simulink model "V1_Pendel"  (R2021a)
settings: Solver=ode3  StartTime=0.0  StopTime=Zeit(end)  FixedStep=0.001  RelTol=1e-3
values from neighbouring files (symbols this model uses):
  Amplitude_rad = (Amplitude/180) * pi    [V1_Schaetzung_d.m]
  d = 0.0042    [V1_Parameter_Stahl_math.m]    (also in V1_Parameter_Stahl_phys.m = 0.0043; V1_Parameter_Styropor_math.m = 0.00019; V1_Parameter_Styropor_phys.m = 0.0018; V1_Schaetzung_d.m = m*g*l*(cos(phi_2) - cos(phi_1))/Integral)
  g = 9.81    [V1_Parameter_Stahl_math.m]    (also in V1_Parameter_Stahl_phys.m; V1_Parameter_Styropor_math.m; V1_Parameter_Styropor_phys.m)
  J = m * l^2    (= 0.503397949)    [V1_Parameter_Stahl_math.m]    (also in V1_Parameter_Stahl_phys.m = 0.512724514275; V1_Parameter_Styropor_math.m = 0.00169341029375; V1_Parameter_Styropor_phys.m = 0.0103382057863)
  l = l_S - s + r_K    (= 0.6005)    [V1_Parameter_Stahl_math.m]    (also in V1_Parameter_Stahl_phys.m = 0.459355833378; V1_Parameter_Styropor_math.m = 0.60025; V1_Parameter_Styropor_phys.m = 0.0522765339967)
  m = m_K    (= 1.396)    [V1_Parameter_Stahl_math.m]    (also in V1_Parameter_Stahl_phys.m = 1.8737; V1_Parameter_Styropor_math.m = 0.0047; V1_Parameter_Styropor_phys.m = 0.4824)
settings Model: Creator=schmi  LastModifiedBy=schmi

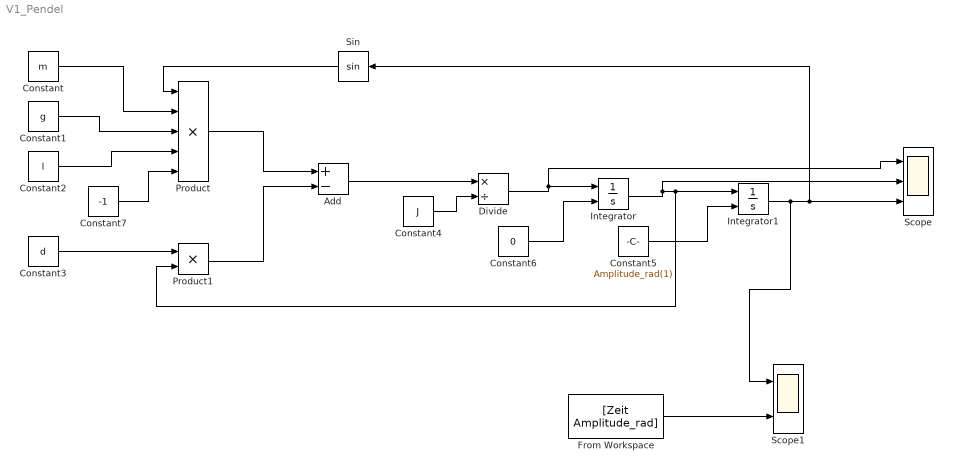
== system V1_Pendel ==
  Add : Sum  Inputs=+-
  Constant : Constant  Value=m
  Constant1 : Constant  Value=g
  Constant2 : Constant  Value=l
  Constant3 : Constant  Value=d
  Constant4 : Constant  Value=J
  Constant5 : Constant  Value=Amplitude_rad(1)
  Constant6 : Constant  Value=0
  Constant7 : Constant  Value=-1
  Divide : Product  Inputs=*/
  From Workspace : FromWorkspace  VariableName=[Zeit Amplitude_rad]
  Integrator : Integrator  InitialConditionSource=external
  Integrator1 : Integrator  InitialConditionSource=external
  Product : Product  Inputs=5
  Product1 : Product
  Scope : Scope  NumInputPorts=3
  Scope1 : Scope  NumInputPorts=2
  Sin : Trigonometry
  wires:
  Add/1 -> Divide/1
  Constant2/1 -> Product/4
  Constant1/1 -> Product/3
  Constant/1 -> Product/2
  Constant3/1 -> Product1/1
  Product1/1 -> Add/2
  Product/1 -> Add/1
  Constant4/1 -> Divide/2
  Divide/1 -> Scope/1, Integrator/1
  Sin/1 -> Product/1
  Integrator/1 -> Scope/2, Product1/2, Integrator1/1
  Constant5/1 -> Integrator1/2
  Constant6/1 -> Integrator/2
  Constant7/1 -> Product/5
  From Workspace/1 -> Scope1/2
  Integrator1/1 -> Scope1/1, Scope/3, Sin/1
